simulink model "System"  (R2020b)
settings: Solver=VariableStepAuto  StartTime=0.0  StopTime=10.0  RelTol=1e-3
settings Model: Creator=Wolflight  LastModifiedBy=Wolflight

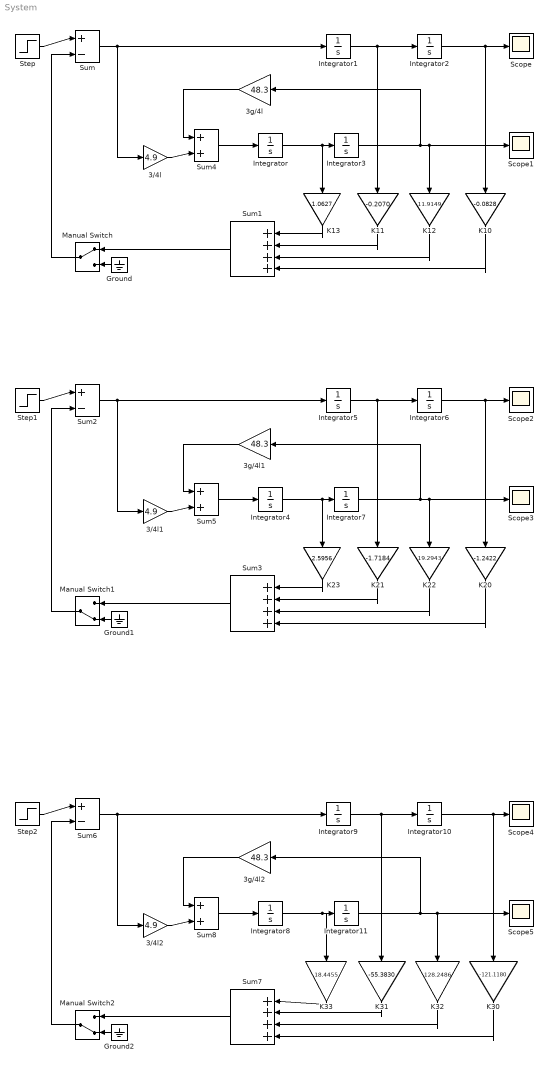
== system System ==
  3/4l : Gain  Gain=4.9
  3/4l1 : Gain  Gain=4.9
  3/4l2 : Gain  Gain=4.9
  3g/4l : Gain  Gain=48.3
  3g/4l1 : Gain  Gain=48.3
  3g/4l2 : Gain  Gain=48.3
  Ground : Ground
  Ground1 : Ground
  Ground2 : Ground
  Integrator{,1..11} (12 alike) : Integrator
  K10 : Gain  Gain=-0.0828
  K11 : Gain  Gain=-0.2070
  K12 : Gain  Gain=11.9149
  K13 : Gain  Gain=1.0627
  K20 : Gain  Gain=-1.2422
  K21 : Gain  Gain=-1.7184
  K22 : Gain  Gain=19.2943
  K23 : Gain  Gain=2.5956
  K30 : Gain  Gain=-121.1180
  K31 : Gain  Gain=-55.3830
  K32 : Gain  Gain=128.2486
  K33 : Gain  Gain=18.4455
  Manual Switch : ManualSwitch
  Manual Switch1 : ManualSwitch  CurrentSetting=0
  Manual Switch2 : ManualSwitch  CurrentSetting=0
  Scope{,1..5} (6 alike) : Scope
  Step : Step  SampleTime=0
  Step1 : Step  SampleTime=0
  Step2 : Step  SampleTime=0
  Sum : Sum  Inputs=|+-
  Sum1 : Sum  Inputs=|++++
  Sum2 : Sum  Inputs=|+-
  Sum3 : Sum  Inputs=|++++
  Sum4 : Sum  Inputs=|++
  Sum5 : Sum  Inputs=|++
  Sum6 : Sum  Inputs=|+-
  Sum7 : Sum  Inputs=|++++
  Sum8 : Sum  Inputs=|++
  wires:
  Step/1 -> Sum/1
  Sum/1 -> 3/4l/1, Integrator1/1
  Integrator1/1 -> K11/1, Integrator2/1
  Integrator2/1 -> K10/1, Scope/1
  3g/4l/1 -> Sum4/1
  3/4l/1 -> Sum4/2
  Sum4/1 -> Integrator/1
  Integrator/1 -> K13/1, Integrator3/1
  Integrator3/1 -> K12/1, Scope1/1, 3g/4l/1
  K13/1 -> Sum1/1
  K11/1 -> Sum1/2
  K12/1 -> Sum1/3
  K10/1 -> Sum1/4
  Sum1/1 -> Manual Switch/1
  Ground/1 -> Manual Switch/2
  Manual Switch/1 -> Sum/2
  Ground1/1 -> Manual Switch1/2
  K21/1 -> Sum3/2
  K23/1 -> Sum3/1
  3/4l1/1 -> Sum5/2
  K20/1 -> Sum3/4
  K22/1 -> Sum3/3
  Integrator4/1 -> K23/1, Integrator7/1
  Integrator7/1 -> K22/1, Scope3/1, 3g/4l1/1
  Sum3/1 -> Manual Switch1/1
  Sum2/1 -> 3/4l1/1, Integrator5/1
  Sum5/1 -> Integrator4/1
  Integrator6/1 -> K20/1, Scope2/1
  3g/4l1/1 -> Sum5/1
  Step1/1 -> Sum2/1
  Integrator5/1 -> K21/1, Integrator6/1
  Manual Switch1/1 -> Sum2/2
  3g/4l2/1 -> Sum8/1
  Step2/1 -> Sum6/1
  Manual Switch2/1 -> Sum6/2
  Integrator10/1 -> K30/1, Scope4/1
  Integrator9/1 -> K31/1, Integrator10/1
  Sum6/1 -> 3/4l2/1, Integrator9/1
  Sum7/1 -> Manual Switch2/1
  Integrator11/1 -> K32/1, Scope5/1, 3g/4l2/1
  Sum8/1 -> Integrator8/1
  Integrator8/1 -> K33/1, Integrator11/1
  K33/1 -> Sum7/1
  K32/1 -> Sum7/3
  K31/1 -> Sum7/2
  3/4l2/1 -> Sum8/2
  K30/1 -> Sum7/4
  Ground2/1 -> Manual Switch2/2
